simulink model "mass_spring_damper"  (R2019b)
settings: Solver=FixedStepAuto  StartTime=0.0  StopTime=50  FixedStep=0.01  RelTol=1e-3
values from neighbouring files (symbols this model uses):
  b = c(2)    [EKF_estimator.m]    (also in EKF_msd_estimator.m = 0.01; KF_estimator.m = 0.01; Linear_regression_parameter_estimator.m = 0.5; convert_model_for_AMPC.m = 0.5)
  k = c(3)    [EKF_estimator.m]    (also in EKF_msd_estimator.m = 5; HAVOK.m = 1.1; KF_estimator.m = 5; Linear_regression_parameter_estimator.m = 5)
  m = size(y_data,1)    [DMDc_param_sweep.m]    (also in EKF_estimator.m = numel(f_x); EKF_msd_estimator.m = numel(f_x); HAVOK.m = 1; HAVOK_param_sweep.m)
  x0 = [0; 0; 0; 0; 0; 1]    [EKF_estimator.m]    (also in EKF_msd_estimator.m = [0; 0]; HAVOK.m = [0.5; 0]; KF_estimator.m = [0; 0]; Linear_regression_state_estimator.m = [0;0;0;0])
libraries: simulink x1
settings Model: Creator=Murray  LastModifiedBy=Murray

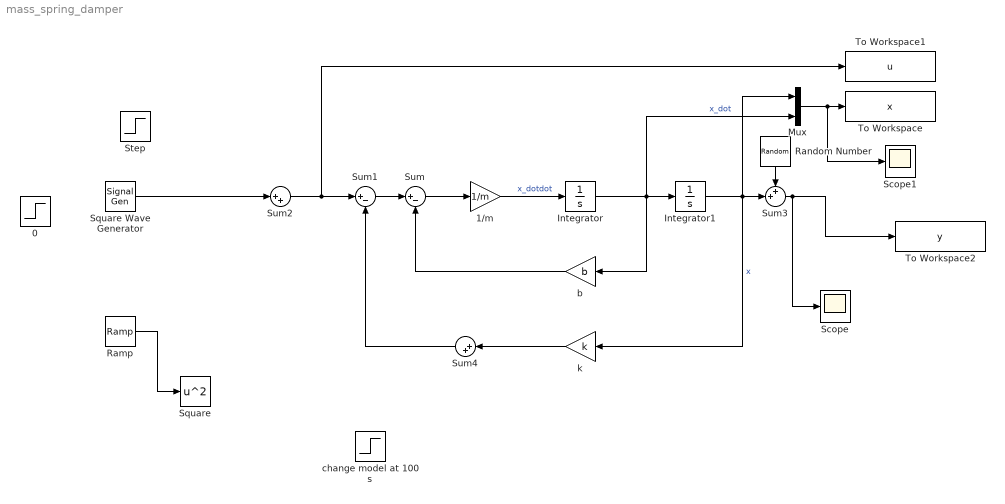
== system mass_spring_damper ==
  0 : Step  Time=0.01  Before=1  After=0  SampleTime=0
  1/m : Gain  Gain=1/m
  Integrator : Integrator  InitialCondition=x0(2)
  Integrator1 : Integrator  InitialCondition=x0(1)
  Mux : Mux  Inputs=2
  Ramp : simulink/Sources/Ramp  slope=1  start=0  InitialOutput=0
  Random Number : RandomNumber  Variance=0.01  SampleTime=0.01
  Scope : Scope
  Scope1 : Scope
  Square : Math  Operator=square  SignedPower=off  SaturateOnIntegerOverflow=on
  Square Wave Generator : SignalGenerator  WaveForm=square  Amplitude=5  Frequency=1/10
  Step : Step  SampleTime=0
  Sum : Sum  Inputs=|+-
  Sum1 : Sum  Inputs=|+-
  Sum2 : Sum  Inputs=|++
  Sum3 : Sum  Inputs=++|
  Sum4 : Sum  Inputs=|++
  To Workspace : ToWorkspace  VariableName=x  SaveFormat=Timeseries  SampleTime=-1
  To Workspace1 : ToWorkspace  VariableName=u  SaveFormat=Timeseries  SampleTime=-1
  To Workspace2 : ToWorkspace  VariableName=y  SaveFormat=Timeseries  SampleTime=-1
  b : Gain  Gain=b
  change model at 100 s : Step  Time=20  SampleTime=0
  k : Gain  Gain=k
  wires:
  1/m/1 -> Integrator/1  "x_dotdot"
  Sum/1 -> 1/m/1
  Integrator/1 -> b/1, Mux/2, Integrator1/1  "x_dot"
  b/1 -> Sum/2
  Sum1/1 -> Sum/1
  Integrator1/1 -> Mux/1, Sum3/2, k/1  "x"
  Sum2/1 -> To Workspace1/1, Sum1/1
  Ramp/1 -> Square/1
  Square Wave Generator/1 -> Sum2/1
  Sum3/1 -> To Workspace2/1, Scope/1
  k/1 -> Sum4/1
  Sum4/1 -> Sum1/2
  Random Number/1 -> Sum3/1
  Mux/1 -> Scope1/1, To Workspace/1
